simulink model "TactileStimEEG_New"  (R2014a)
settings: Solver=FixedStepDiscrete  StartTime=0.0  StopTime=inf  RelTol=1e-3
model workspace (MAT data in the model file):
  local_ip = 2130706433
  local_port = 50224
  host_ip = 2130706433
  host_port = 50223
  sample_rate = 500
  num_samples = 8
  num_en_channels = 16
  en_add_channels = 127
  cfg_native : struct (value not decoded)
  serial_number = 'NB-2015.02.21'
undefined symbols (not defined in the file or in its folder): NB
libraries: gNautilusLib x1, gNautilusTools x1, gtecHighspeedLib x1
settings Model: Creator=Maresch  LastModifiedBy=ENL
settings DataIOCC: LimitDataPoints=off  SignalLoggingSaveFormat=ModelDataLogs  SaveOutput=off  SignalLogging=off  SaveTime=off
settings OptimizationCC: ExpressionDepthLimit=2147483647  InitFltsAndDblsToZero=on  OptimizeModelRefInitCode=on
settings DebuggingCC: SaveWithParameterizedLinksMsg=none  UnderspecifiedInitializationDetection=Classic  SignalResolutionControl=TryResolveAllWithWarning  MultiTaskDSMMsg=warning  MultiTaskCondExecSysMsg=none  IntegerOverflowMsg=none  FcnCallInpInsideContextMsg=UseLocalSettings  UnconnectedInputMsg=none  UnconnectedOutputMsg=none  StateNameClashWarn=warning
settings HardwareCC: ProdIntDivRoundTo=Floor  ProdEndianess=LittleEndian  ProdHWDeviceType=32-bit xPC Target (Intel Pentium)  TargetHWDeviceType=32-bit Generic
settings RTWCC: SystemTargetFile=ccslink_ert.tlc  GenCodeOnly=on  GenerateMakefile=off  TemplateMakefile=ccslink_ert.tmf  Description=Link for CCS (ERT) code generation for TMS320(TM) DSP platforms  ProcessScript=ccslink_ert_make_rtw_hook  IncludeERTFirstTime=on
settings CodeAppCC: IgnoreCustomStorageClasses=off
settings TargetCC: CompOptLevelCompliant=off  ERTCustomFileBanners=on  MatFileLogging=on  SupportContinuousTime=off  SupportNonInlinedSFcns=off  EnableShiftOperators=on

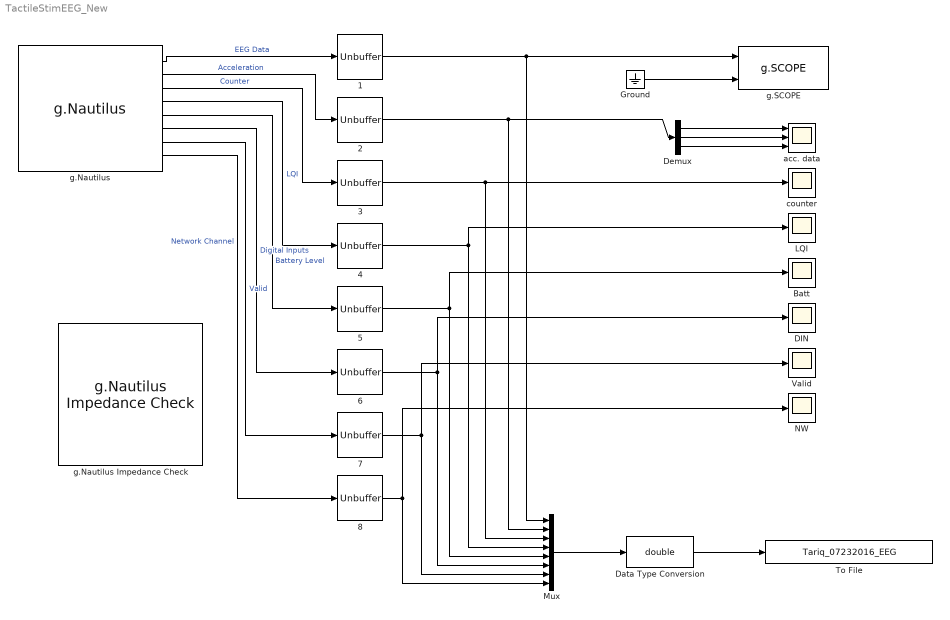
== system TactileStimEEG_New ==
  {1..8} (8 alike) : Unbuffer  SampleBasedProcessing=Same as frame based
  Batt : Scope
      settings: SaveName=ScopeData3
  DIN : Scope
      settings: SaveName=ScopeData4
  Data Type Conversion : DataTypeConversion  OutDataTypeStr=double
  Demux : Demux  Outputs=3
  Ground : Ground
  LQI : Scope
      settings: SaveName=ScopeData2
  Mux : Mux  Inputs=8
  NW : Scope
      settings: SaveName=ScopeData6
  To File : ToFile  Filename=Tariq_07232016_EEG  MatrixName=y
  Valid : Scope
      settings: SaveName=ScopeData5
  acc. data : Scope  NumInputPorts=3
      settings: TimeRange=60  YMin=-6~-6~-2  YMax=6~6~2
  counter : Scope
  g.Nautilus : gNautilusLib/g.Nautilus  Tag=g.Nautilus  Description=Operates a g.Nautilus device and provides acquired data on its outputs.  sample_rate=500  local_ip=2130706433  local_port=50224  host_ip=2130706433  host_port=50223  serial_number=NB-2015.02.21  num_samples=8  num_en_channels=16  add_channels=127
  g.Nautilus Impedance Check : gNautilusTools/g.Nautilus Impedance Check
  g.SCOPE : gtecHighspeedLib/g.SCOPE
  wires:
  g.Nautilus/1 -> 1/1  "EEG Data"
  g.Nautilus/2 -> 2/1  "Acceleration"
  g.Nautilus/3 -> 3/1  "Counter"
  g.Nautilus/4 -> 4/1  "LQI"
  g.Nautilus/5 -> 5/1  "Battery Level"
  g.Nautilus/6 -> 6/1  "Digital Inputs"
  g.Nautilus/7 -> 7/1  "Valid"
  g.Nautilus/8 -> 8/1  "Network Channel"
  Data Type Conversion/1 -> To File/1
  Mux/1 -> Data Type Conversion/1
  7/1 -> Valid/1, Mux/7
  Demux/2 -> acc. data/2
  Ground/1 -> g.SCOPE/2
  Demux/1 -> acc. data/1
  Demux/3 -> acc. data/3
  1/1 -> Mux/1, g.SCOPE/1
  2/1 -> Mux/2, Demux/1
  3/1 -> counter/1, Mux/3
  4/1 -> LQI/1, Mux/4
  5/1 -> Mux/5, Batt/1
  6/1 -> Mux/6, DIN/1
  8/1 -> Mux/8, NW/1
